simulink model "IEEE9Bus_new"  (R2020b)
settings: Solver=ode23tb  StartTime=0.0  StopTime=0.2  MaxStep=50e-6  RelTol=1e-3  EnableMultiTasking=on
values from neighbouring files (symbols this model uses):
  x = 50    [Xconst.m]    (also in wt_new.m = p(i))
libraries: powerlib x49
settings Model: Creator=salam  LastModifiedBy=Lenovo G50-80
settings DataIOCC: ReturnWorkspaceOutputs=off
settings DebuggingCC: ArithmeticOperatorsInVariantConditions=warning
settings SFSimCC: CustomCodeUndefinedFunction=UseInterfaceOnly
settings CodeAppCC: StateflowObjectComments=on
settings SimscapeCC: SimscapeNormalizeSystem=off

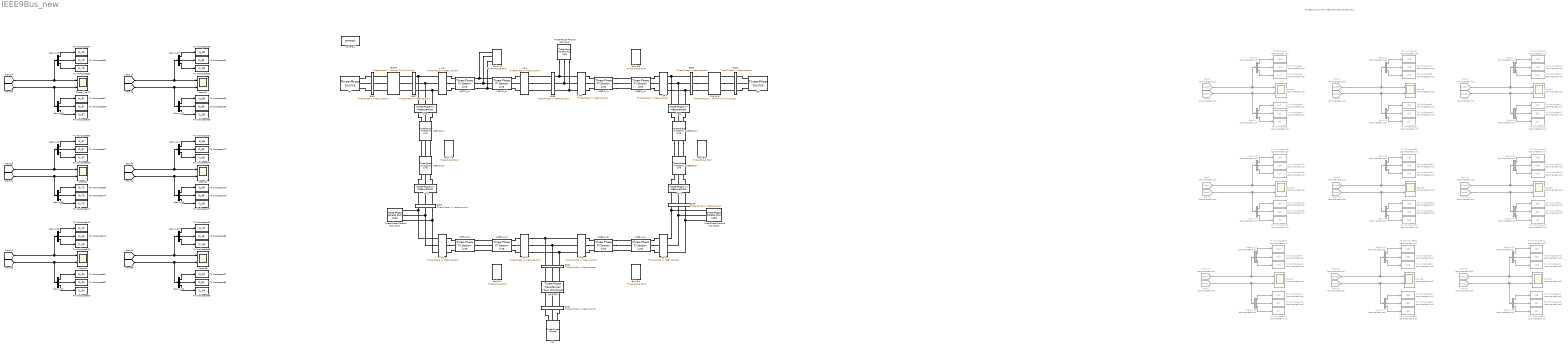
== system IEEE9Bus_new ==
  note: Voltage and Current Measurements at each Bus
  + 46 - : powerlib/Measurements/Three-Phase V-I Measurement  VoltageMeasurement=no  SetLabelV=on  LabelV=Vabc_78  Vpu=on  VpuLL=off  CurrentMeasurement=yes  SetLabelI=on  LabelI=Iabc_46  Ipu=off  Pbase=100e6  Vbase=230e3  OutputType=Complex  PhasorSimulation=off  PSBequivalent=0
  + 54 - : powerlib/Measurements/Three-Phase V-I Measurement  VoltageMeasurement=no  SetLabelV=on  LabelV=Vabc_78  Vpu=on  VpuLL=off  CurrentMeasurement=yes  SetLabelI=on  LabelI=Iabc_54  Ipu=off  Pbase=100e6  Vbase=230e3  OutputType=Complex  PhasorSimulation=off  PSBequivalent=0
  + 75 - : powerlib/Measurements/Three-Phase V-I Measurement  VoltageMeasurement=no  SetLabelV=on  LabelV=Vabc_87  Vpu=on  VpuLL=off  CurrentMeasurement=yes  SetLabelI=on  LabelI=Iabc_75  Ipu=off  Pbase=100e6  Vbase=230e3  OutputType=Complex  PhasorSimulation=off  PSBequivalent=0
  + 78 - : powerlib/Measurements/Three-Phase V-I Measurement  VoltageMeasurement=no  SetLabelV=on  LabelV=Vabc_78  Vpu=on  VpuLL=off  CurrentMeasurement=yes  SetLabelI=on  LabelI=Iabc_78  Ipu=off  Pbase=100e6  Vbase=230e3  OutputType=Complex  PhasorSimulation=off  PSBequivalent=0
  + 89 - : powerlib/Measurements/Three-Phase V-I Measurement  VoltageMeasurement=no  SetLabelV=on  LabelV=Vabc_78  Vpu=on  VpuLL=off  CurrentMeasurement=yes  SetLabelI=on  LabelI=Iabc_89  Ipu=off  Pbase=100e6  Vbase=230e3  OutputType=Complex  PhasorSimulation=off  PSBequivalent=0
  + 96 - : powerlib/Measurements/Three-Phase V-I Measurement  VoltageMeasurement=no  SetLabelV=on  LabelV=Vabc_87  Vpu=on  VpuLL=off  CurrentMeasurement=yes  SetLabelI=on  LabelI=Iabc_96  Ipu=off  Pbase=100e6  Vbase=230e3  OutputType=Complex  PhasorSimulation=off  PSBequivalent=0
  - 46 + : powerlib/Measurements/Three-Phase V-I Measurement  VoltageMeasurement=no  SetLabelV=on  LabelV=Vabc_87  Vpu=on  VpuLL=off  CurrentMeasurement=yes  SetLabelI=on  LabelI=Iabc_64  Ipu=off  Pbase=100e6  Vbase=230e3  OutputType=Complex  PhasorSimulation=off  PSBequivalent=0
  - 54 + : powerlib/Measurements/Three-Phase V-I Measurement  VoltageMeasurement=no  SetLabelV=on  LabelV=Vabc_87  Vpu=on  VpuLL=off  CurrentMeasurement=yes  SetLabelI=on  LabelI=Iabc_45  Ipu=off  Pbase=100e6  Vbase=230e3  OutputType=Complex  PhasorSimulation=off  PSBequivalent=0
  - 75 + : powerlib/Measurements/Three-Phase V-I Measurement  VoltageMeasurement=no  SetLabelV=on  LabelV=Vabc_87  Vpu=on  VpuLL=off  CurrentMeasurement=yes  SetLabelI=on  LabelI=Iabc_57  Ipu=off  Pbase=100e6  Vbase=230e3  OutputType=Complex  PhasorSimulation=off  PSBequivalent=0
  - 78 + : powerlib/Measurements/Three-Phase V-I Measurement  VoltageMeasurement=no  SetLabelV=on  LabelV=Vabc_87  Vpu=on  VpuLL=off  CurrentMeasurement=yes  SetLabelI=on  LabelI=Iabc_87  Ipu=off  Pbase=100e6  Vbase=230e3  OutputType=Complex  PhasorSimulation=off  PSBequivalent=0
  - 89 + : powerlib/Measurements/Three-Phase V-I Measurement  VoltageMeasurement=no  SetLabelV=on  LabelV=Vabc_87  Vpu=on  VpuLL=off  CurrentMeasurement=yes  SetLabelI=on  LabelI=Iabc_98  Ipu=off  Pbase=100e6  Vbase=230e3  OutputType=Complex  PhasorSimulation=off  PSBequivalent=0
  - 96 + : powerlib/Measurements/Three-Phase V-I Measurement  VoltageMeasurement=no  SetLabelV=on  LabelV=Vabc_87  Vpu=on  VpuLL=off  CurrentMeasurement=yes  SetLabelI=on  LabelI=Iabc_69  Ipu=off  Pbase=100e6  Vbase=230e3  OutputType=Complex  PhasorSimulation=off  PSBequivalent=0
  16.5/230 : powerlib/Elements/Three-Phase Transformer (Two Windings)  Winding1Connection=Yg  Winding2Connection=Yg  CoreType=Three single-phase transformers  SetSaturation=off  Hysteresis=off  DataFile='hysteresis'  SetInitialFlux=off  Measurements=None  UNITS=pu  NominalPower=[ 100e6 , 50 ]  Winding1=[ 24e3 , 1e-6, 0 ]  Winding2=[ 230e3 ,1e-6, 0.0576 ]  Rm=500  Lm=500  L0=0.5  Saturation=[ 0,0 ; 0.0024,1.2 ; 1.0,1.52 ]  InitialFluxes=[ 0.8 , -0.8 , 0.7 ]  BreakLoop=off  DiscreteSolver=Trapezoidal iterative  DataType=off  TransfoNumber=1
  18/230 : powerlib/Elements/Three-Phase Transformer (Two Windings)  Winding1Connection=Yg  Winding2Connection=Yg  CoreType=Three single-phase transformers  SetSaturation=off  Hysteresis=off  DataFile='hysteresis'  SetInitialFlux=off  Measurements=None  UNITS=pu  NominalPower=[ 100e6 , 50 ]  Winding1=[ 18e3 , 1e-6 , 0]  Winding2=[ 230e3 , 1e-6, 0.0625 ]  Rm=500  Lm=500  L0=0.5  Saturation=[ 0,0 ; 0.0024,1.2 ; 1.0,1.52 ]  InitialFluxes=[ 0.8 , -0.8 , 0.7 ]  BreakLoop=off  DiscreteSolver=Trapezoidal iterative  DataType=off  TransfoNumber=1
  230/13.8 : powerlib/Elements/Three-Phase Transformer (Two Windings)  Winding1Connection=Yg  Winding2Connection=Yg  CoreType=Three single-phase transformers  SetSaturation=off  Hysteresis=off  DataFile='hysteresis'  SetInitialFlux=off  Measurements=None  UNITS=pu  NominalPower=[ 100e6 , 50 ]  Winding1=[ 13.8e3 , 1e-6 , 0 ]  Winding2=[ 230e3 , 1e-6, 0.0586 ]  Rm=500  Lm=500  L0=0.5  Saturation=[ 0,0 ; 0.0024,1.2 ; 1.0,1.52 ]  InitialFluxes=[ 0.8 , -0.8 , 0.7 ]  BreakLoop=off  DiscreteSolver=Trapezoidal iterative  DataType=off  TransfoNumber=1
  BUS1 : powerlib/Measurements/Three-Phase V-I Measurement  VoltageMeasurement=phase-to-ground  SetLabelV=on  LabelV=Vabc1  Vpu=off  VpuLL=off  CurrentMeasurement=yes  SetLabelI=on  LabelI=Iabc1  Ipu=off  Pbase=100e6  Vbase=500e3  OutputType=Complex  PhasorSimulation=off  PSBequivalent=0
  BUS2 : powerlib/Measurements/Three-Phase V-I Measurement  VoltageMeasurement=phase-to-ground  SetLabelV=on  LabelV=Vabc2  Vpu=off  VpuLL=off  CurrentMeasurement=yes  SetLabelI=on  LabelI=Iabc2  Ipu=off  Pbase=100e6  Vbase=500e3  OutputType=Complex  PhasorSimulation=off  PSBequivalent=0
  BUS3 : powerlib/Measurements/Three-Phase V-I Measurement  VoltageMeasurement=phase-to-ground  SetLabelV=on  LabelV=Vabc3  Vpu=off  VpuLL=off  CurrentMeasurement=yes  SetLabelI=on  LabelI=Iabc3  Ipu=off  Pbase=100e6  Vbase=500e3  OutputType=Complex  PhasorSimulation=off  PSBequivalent=0
  BUS4 : powerlib/Measurements/Three-Phase V-I Measurement  VoltageMeasurement=phase-to-ground  SetLabelV=on  LabelV=Vabc4  Vpu=off  VpuLL=off  CurrentMeasurement=yes  SetLabelI=on  LabelI=Iabc4  Ipu=off  Pbase=100e6  Vbase=500e3  OutputType=Complex  PhasorSimulation=off  PSBequivalent=0
  BUS5 : powerlib/Measurements/Three-Phase V-I Measurement  VoltageMeasurement=phase-to-ground  SetLabelV=on  LabelV=Vabc5  Vpu=off  VpuLL=off  CurrentMeasurement=yes  SetLabelI=on  LabelI=Iabc5  Ipu=off  Pbase=100e6  Vbase=500e3  OutputType=Complex  PhasorSimulation=off  PSBequivalent=0
  BUS6 : powerlib/Measurements/Three-Phase V-I Measurement  VoltageMeasurement=phase-to-ground  SetLabelV=on  LabelV=Vabc6  Vpu=off  VpuLL=off  CurrentMeasurement=yes  SetLabelI=on  LabelI=Iabc6  Ipu=off  Pbase=100e6  Vbase=500e3  OutputType=Complex  PhasorSimulation=off  PSBequivalent=0
  BUS7 : powerlib/Measurements/Three-Phase V-I Measurement  VoltageMeasurement=phase-to-ground  SetLabelV=on  LabelV=Vabc7  Vpu=off  VpuLL=off  CurrentMeasurement=yes  SetLabelI=on  LabelI=Iabc7  Ipu=off  Pbase=100e6  Vbase=500e3  OutputType=Complex  PhasorSimulation=off  PSBequivalent=0
  BUS8 : powerlib/Measurements/Three-Phase V-I Measurement  VoltageMeasurement=phase-to-ground  SetLabelV=on  LabelV=Vabc8  Vpu=off  VpuLL=off  CurrentMeasurement=yes  SetLabelI=on  LabelI=Iabc8  Ipu=off  Pbase=100e6  Vbase=500e3  OutputType=Complex  PhasorSimulation=off  PSBequivalent=0
  BUS9 : powerlib/Measurements/Three-Phase V-I Measurement  VoltageMeasurement=phase-to-ground  SetLabelV=on  LabelV=Vabc9  Vpu=off  VpuLL=off  CurrentMeasurement=yes  SetLabelI=on  LabelI=Iabc9  Ipu=off  Pbase=100e6  Vbase=500e3  OutputType=Complex  PhasorSimulation=off  PSBequivalent=0
  Demux{,1..17} (18 alike) : Demux  Commented=on  Outputs=3
  Demux{18..29} (12 alike) : Demux  Outputs=3
  From1 : From  Commented=on  GotoTag=Vabc1  TagVisibility=global
  From10 : From  Commented=on  GotoTag=Iabc5  TagVisibility=global
  From11 : From  Commented=on  GotoTag=Vabc6  TagVisibility=global
  From12 : From  Commented=on  GotoTag=Iabc6  TagVisibility=global
  From13 : From  Commented=on  GotoTag=Iabc8  TagVisibility=global
  From14 : From  Commented=on  GotoTag=Vabc9  TagVisibility=global
  From15 : From  Commented=on  GotoTag=Iabc9  TagVisibility=global
  From16 : From  Commented=on  GotoTag=Vabc7  TagVisibility=global
  From17 : From  Commented=on  GotoTag=Iabc7  TagVisibility=global
  From18 : From  Commented=on  GotoTag=Vabc8  TagVisibility=global
  From2 : From  Commented=on  GotoTag=Iabc1  TagVisibility=global
  From3 : From  Commented=on  GotoTag=Vabc2  TagVisibility=global
  From4 : From  Commented=on  GotoTag=Iabc2  TagVisibility=global
  From5 : From  Commented=on  GotoTag=Vabc3  TagVisibility=global
  From6 : From  Commented=on  GotoTag=Iabc3  TagVisibility=global
  From7 : From  Commented=on  GotoTag=Vabc4  TagVisibility=global
  From8 : From  Commented=on  GotoTag=Iabc4  TagVisibility=global
  From9 : From  Commented=on  GotoTag=Vabc5  TagVisibility=global
  G1 : powerlib/Electrical Sources/Three-Phase Source  InternalConnection=Yg  VoltagePhases=off  Voltage=16500  PhaseAngle=0  Voltage_phases=[25e3 25e3 25e3]/sqrt(3)  PhaseAngles_phases=[0 -120 +120]  Frequency=50  NonIdealSource=on  SpecifyImpedance=off  Resistance=0.8929  Inductance=16.58e-3  ShortCircuitLevel=247.5e6  BaseVoltage=16.5e3  XRratio=100000  BusType=swing  Pref=10e3  Qref=0  Prefabc=[10e3, 10e3, 10e3]  Qrefabc=[0, 0, 0]  Qmin=-inf  Qmax=inf
  G2 : powerlib/Electrical Sources/Three-Phase Source  InternalConnection=Yg  VoltagePhases=off  Voltage=18e3  PhaseAngle=0  Voltage_phases=[25e3 25e3 25e3]/sqrt(3)  PhaseAngles_phases=[0 -120 +120]  Frequency=50  NonIdealSource=on  SpecifyImpedance=off  Resistance=0.8929  Inductance=16.58e-3  ShortCircuitLevel=192e6  BaseVoltage=18e3  XRratio=100000  BusType=PV  Pref=163e6  Qref=0  Prefabc=[10e3, 10e3, 10e3]  Qrefabc=[0, 0, 0]  Qmin=-inf  Qmax=inf
  G3 : powerlib/Electrical Sources/Three-Phase Source  InternalConnection=Yg  VoltagePhases=off  Voltage=13800  PhaseAngle=0  Voltage_phases=[25e3 25e3 25e3]/sqrt(3)  PhaseAngles_phases=[0 -120 +120]  Frequency=50  NonIdealSource=on  SpecifyImpedance=off  Resistance=0.8929  Inductance=16.58e-3  ShortCircuitLevel=128e6  BaseVoltage=13.8e3  XRratio=100000  BusType=PV  Pref=85e6  Qref=0  Prefabc=[10e3, 10e3, 10e3]  Qrefabc=[0, 0, 0]  Qmin=-inf  Qmax=inf
  LINE5-4_(1) : powerlib/Elements/Three-Phase PI Section Line  LConnTagsString=a|b|c  RConnTagsString=A|B|C  Length=47.38  Frequency=50  Resistances=[ 0.01273 0.3864]  Inductances="[ 0.9337e-3  4.1264e-3]"  Capacitances=[12.74e-9 7.751e-9]
  LINE5-4_(2) : powerlib/Elements/Three-Phase PI Section Line  LConnTagsString=a|b|c  RConnTagsString=A|B|C  Length=50  Frequency=50  Resistances=[ 0.01273 0.3864]  Inductances="[ 0.9337e-3  4.1264e-3]"  Capacitances=[12.74e-9 7.751e-9]
  LINE6-4_(1) : powerlib/Elements/Three-Phase PI Section Line  LConnTagsString=a|b|c  RConnTagsString=A|B|C  Length=45.99  Frequency=50  Resistances=[ 0.01273 0.3864]  Inductances="[ 0.9337e-3  4.1264e-3]"  Capacitances=[12.74e-9 7.751e-9]
  LINE6-4_(2) : powerlib/Elements/Three-Phase PI Section Line  LConnTagsString=a|b|c  RConnTagsString=A|B|C  Length=50  Frequency=50  Resistances=[ 0.01273 0.3864]  Inductances="[ 0.9337e-3  4.1264e-3]"  Capacitances=[12.74e-9 7.751e-9]
  LINE7-5_(1) : powerlib/Elements/Three-Phase PI Section Line  LConnTagsString=a|b|c  RConnTagsString=A|B|C  Length=100  Frequency=50  Resistances=[ 0.01273 0.3864]  Inductances="[ 0.9337e-3  4.1264e-3]"  Capacitances=[12.74e-9 7.751e-9]
  LINE7-5_(2) : powerlib/Elements/Three-Phase PI Section Line  LConnTagsString=a|b|c  RConnTagsString=A|B|C  Length=76.71  Frequency=50  Resistances=[ 0.01273 0.3864]  Inductances="[ 0.9337e-3  4.1264e-3]"  Capacitances=[12.74e-9 7.751e-9]
  LINE7-8_(1) : powerlib/Elements/Three-Phase PI Section Line  LConnTagsString=a|b|c  RConnTagsString=A|B|C  Length=98.95*x*.01+.001  Frequency=50  Resistances=[ 0.01273 0.3864]  Inductances="[ 0.9337e-3  4.1264e-3]"  Capacitances=[12.74e-9 7.751e-9]
  LINE7-8_(2) : powerlib/Elements/Three-Phase PI Section Line  LConnTagsString=a|b|c  RConnTagsString=A|B|C  Length=98.95*(1-x*.01)+.001  Frequency=50  Resistances=[ 0.01273 0.3864]  Inductances="[ 0.9337e-3  4.1264e-3]"  Capacitances=[12.74e-9 7.751e-9]
  LINE8-9_(1) : powerlib/Elements/Three-Phase PI Section Line  LConnTagsString=a|b|c  RConnTagsString=A|B|C  Length=65.56  Frequency=50  Resistances=[ 0.01273 0.3864]  Inductances="[ 0.9337e-3  4.1264e-3]"  Capacitances=[12.74e-9 7.751e-9]
  LINE8-9_(2) : powerlib/Elements/Three-Phase PI Section Line  LConnTagsString=a|b|c  RConnTagsString=A|B|C  Length=50  Frequency=50  Resistances=[ 0.01273 0.3864]  Inductances="[ 0.9337e-3  4.1264e-3]"  Capacitances=[12.74e-9 7.751e-9]
  LINE9-6_(1) : powerlib/Elements/Three-Phase PI Section Line  LConnTagsString=a|b|c  RConnTagsString=A|B|C  Length=100  Frequency=50  Resistances=[ 0.01273 0.3864]  Inductances="[ 0.9337e-3  4.1264e-3]"  Capacitances=[12.74e-9 7.751e-9]
  LINE9-6_(2) : powerlib/Elements/Three-Phase PI Section Line  LConnTagsString=a|b|c  RConnTagsString=A|B|C  Length=96.41  Frequency=50  Resistances=[ 0.01273 0.3864]  Inductances="[ 0.9337e-3  4.1264e-3]"  Capacitances=[12.74e-9 7.751e-9]
  Scope{1..9} (9 alike) : Scope  Commented=on  NumInputPorts=2
  Scope{11..15} (5 alike) : Scope  NumInputPorts=2
  Scope_line78 : Scope  NumInputPorts=2
  Three-Phase Parallel RLC Load : powerlib/Elements/Three-Phase Parallel RLC Load  LConnTagsString=A|B|C  Configuration=Y (grounded)  NominalVoltage=230000  Vabc=[1e3 1e3 1e3]  Vabcp=[1e3 1e3 1e3]  NominalFrequency=50  UnbalancedPower=off  ActivePower=100e6  InductivePower=35e6  CapacitivePower=0  Pabc=[10e3 9e3 11e3]  QLabc=[100 90 110]  QCabc=[100 90 110]  Pabcp=[10e3 9e3 11e3]  QLabcp=[100 90 110]  QCabcp=[100 90 110]  Measurements=None  LoadType=constant Z
  Three-Phase Parallel RLC Load1 : powerlib/Elements/Three-Phase Parallel RLC Load  LConnTagsString=A|B|C  Configuration=Y (grounded)  NominalVoltage=230000  Vabc=[1e3 1e3 1e3]  Vabcp=[1e3 1e3 1e3]  NominalFrequency=50  UnbalancedPower=off  ActivePower=125e6  InductivePower=50e6  CapacitivePower=0  Pabc=[10e3 9e3 11e3]  QLabc=[100 90 110]  QCabc=[100 90 110]  Pabcp=[10e3 9e3 11e3]  QLabcp=[100 90 110]  QCabcp=[100 90 110]  Measurements=None  LoadType=constant Z
  Three-Phase Parallel RLC Load2 : powerlib/Elements/Three-Phase Parallel RLC Load  LConnTagsString=A|B|C  Configuration=Y (grounded)  NominalVoltage=230000  Vabc=[1e3 1e3 1e3]  Vabcp=[1e3 1e3 1e3]  NominalFrequency=50  UnbalancedPower=off  ActivePower=90e6  InductivePower=30e6  CapacitivePower=0  Pabc=[10e3 9e3 11e3]  QLabc=[100 90 110]  QCabc=[100 90 110]  Pabcp=[10e3 9e3 11e3]  QLabcp=[100 90 110]  QCabcp=[100 90 110]  Measurements=None  LoadType=constant Z
  To Workspace : ToWorkspace  Commented=on  VariableName=Va1  SampleTime=-1
  To Workspace1 : ToWorkspace  Commented=on  VariableName=Vb1  SampleTime=-1
  To Workspace10 : ToWorkspace  Commented=on  VariableName=Ib2  SampleTime=-1
  To Workspace11 : ToWorkspace  Commented=on  VariableName=Ic2  SampleTime=-1
  To Workspace12 : ToWorkspace  Commented=on  VariableName=Ib3  SampleTime=-1
  To Workspace13 : ToWorkspace  Commented=on  VariableName=Ic3  SampleTime=-1
  To Workspace14 : ToWorkspace  Commented=on  VariableName=Va3  SampleTime=-1
  To Workspace15 : ToWorkspace  Commented=on  VariableName=Vb3  SampleTime=-1
  To Workspace16 : ToWorkspace  Commented=on  VariableName=Vc3  SampleTime=-1
  To Workspace17 : ToWorkspace  Commented=on  VariableName=Ia3  SampleTime=-1
  To Workspace18 : ToWorkspace  Commented=on  VariableName=Va4  SampleTime=-1
  To Workspace19 : ToWorkspace  Commented=on  VariableName=Vb4  SampleTime=-1
  To Workspace2 : ToWorkspace  Commented=on  VariableName=Vc1  SampleTime=-1
  To Workspace20 : ToWorkspace  Commented=on  VariableName=Ib5  SampleTime=-1
  To Workspace21 : ToWorkspace  Commented=on  VariableName=Ic5  SampleTime=-1
  To Workspace22 : ToWorkspace  Commented=on  VariableName=Ib6  SampleTime=-1
  To Workspace23 : ToWorkspace  Commented=on  VariableName=Ic6  SampleTime=-1
  To Workspace24 : ToWorkspace  Commented=on  VariableName=Va6  SampleTime=-1
  To Workspace25 : ToWorkspace  Commented=on  VariableName=Vb6  SampleTime=-1
  To Workspace26 : ToWorkspace  Commented=on  VariableName=Vc6  SampleTime=-1
  To Workspace27 : ToWorkspace  Commented=on  VariableName=Ia6  SampleTime=-1
  To Workspace28 : ToWorkspace  Commented=on  VariableName=Vc4  SampleTime=-1
  To Workspace29 : ToWorkspace  Commented=on  VariableName=Ia4  SampleTime=-1
  To Workspace3 : ToWorkspace  Commented=on  VariableName=Ia1  SampleTime=-1
  To Workspace30 : ToWorkspace  Commented=on  VariableName=Ib4  SampleTime=-1
  To Workspace31 : ToWorkspace  Commented=on  VariableName=Ic4  SampleTime=-1
  To Workspace32 : ToWorkspace  Commented=on  VariableName=Va5  SampleTime=-1
  To Workspace33 : ToWorkspace  Commented=on  VariableName=Vb5  SampleTime=-1
  To Workspace34 : ToWorkspace  Commented=on  VariableName=Vc5  SampleTime=-1
  To Workspace35 : ToWorkspace  Commented=on  VariableName=Ia5  SampleTime=-1
  To Workspace36 : ToWorkspace  Commented=on  VariableName=Va7  SampleTime=-1
  To Workspace37 : ToWorkspace  Commented=on  VariableName=Vb7  SampleTime=-1
  To Workspace38 : ToWorkspace  Commented=on  VariableName=Ib8  SampleTime=-1
  To Workspace39 : ToWorkspace  Commented=on  VariableName=Ic8  SampleTime=-1
  To Workspace4 : ToWorkspace  Commented=on  VariableName=Ib1  SampleTime=-1
  To Workspace40 : ToWorkspace  Commented=on  VariableName=Ib9  SampleTime=-1
  To Workspace41 : ToWorkspace  Commented=on  VariableName=Ic9  SampleTime=-1
  To Workspace42 : ToWorkspace  Commented=on  VariableName=Va9  SampleTime=-1
  To Workspace43 : ToWorkspace  Commented=on  VariableName=Vb9  SampleTime=-1
  To Workspace44 : ToWorkspace  Commented=on  VariableName=Vc9  SampleTime=-1
  To Workspace45 : ToWorkspace  Commented=on  VariableName=Ia9  SampleTime=-1
  To Workspace46 : ToWorkspace  Commented=on  VariableName=Vc7  SampleTime=-1
  To Workspace47 : ToWorkspace  Commented=on  VariableName=Ia7  SampleTime=-1
  To Workspace48 : ToWorkspace  Commented=on  VariableName=Ib7  SampleTime=-1
  To Workspace49 : ToWorkspace  Commented=on  VariableName=Ic7  SampleTime=-1
  To Workspace5 : ToWorkspace  Commented=on  VariableName=Ic1  SampleTime=-1
  To Workspace50 : ToWorkspace  Commented=on  VariableName=Va8  SampleTime=-1
  To Workspace51 : ToWorkspace  Commented=on  VariableName=Vb8  SampleTime=-1
  To Workspace52 : ToWorkspace  Commented=on  VariableName=Vc8  SampleTime=-1
  To Workspace53 : ToWorkspace  Commented=on  VariableName=Ia8  SampleTime=-1
  To Workspace54 : ToWorkspace  VariableName=Ia_78  SampleTime=-1
  To Workspace55 : ToWorkspace  VariableName=Ib_78  SampleTime=-1
  To Workspace56 : ToWorkspace  VariableName=Ic_78  SampleTime=-1
  To Workspace57 : ToWorkspace  VariableName=Ia_87  SampleTime=-1
  To Workspace58 : ToWorkspace  VariableName=Ib_87  SampleTime=-1
  To Workspace59 : ToWorkspace  VariableName=Ic_87  SampleTime=-1
  To Workspace6 : ToWorkspace  Commented=on  VariableName=Va2  SampleTime=-1
  To Workspace60 : ToWorkspace  VariableName=Ia_89  SampleTime=-1
  To Workspace61 : ToWorkspace  VariableName=Ib_89  SampleTime=-1
  To Workspace62 : ToWorkspace  VariableName=Ic_89  SampleTime=-1
  To Workspace63 : ToWorkspace  VariableName=Ia_98  SampleTime=-1
  To Workspace64 : ToWorkspace  VariableName=Ib_98  SampleTime=-1
  To Workspace65 : ToWorkspace  VariableName=Ic_98  SampleTime=-1
  To Workspace66 : ToWorkspace  VariableName=Ia_57  SampleTime=-1
  To Workspace67 : ToWorkspace  VariableName=Ib_57  SampleTime=-1
  To Workspace68 : ToWorkspace  VariableName=Ic_57  SampleTime=-1
  To Workspace69 : ToWorkspace  VariableName=Ia_75  SampleTime=-1
  To Workspace7 : ToWorkspace  Commented=on  VariableName=Vb2  SampleTime=-1
  To Workspace70 : ToWorkspace  VariableName=Ib_75  SampleTime=-1
  To Workspace71 : ToWorkspace  VariableName=Ic_75  SampleTime=-1
  To Workspace72 : ToWorkspace  VariableName=Ia_69  SampleTime=-1
  To Workspace73 : ToWorkspace  VariableName=Ib_69  SampleTime=-1
  To Workspace74 : ToWorkspace  VariableName=Ic_69  SampleTime=-1
  To Workspace75 : ToWorkspace  VariableName=Ia_96  SampleTime=-1
  To Workspace76 : ToWorkspace  VariableName=Ib_96  SampleTime=-1
  To Workspace77 : ToWorkspace  VariableName=Ic_96  SampleTime=-1
  To Workspace78 : ToWorkspace  VariableName=Ia_45  SampleTime=-1
  To Workspace79 : ToWorkspace  VariableName=Ib_45  SampleTime=-1
  To Workspace8 : ToWorkspace  Commented=on  VariableName=Vc2  SampleTime=-1
  To Workspace80 : ToWorkspace  VariableName=Ic_45  SampleTime=-1
  To Workspace81 : ToWorkspace  VariableName=Ia_54  SampleTime=-1
  To Workspace82 : ToWorkspace  VariableName=Ib_54  SampleTime=-1
  To Workspace83 : ToWorkspace  VariableName=Ic_54  SampleTime=-1
  To Workspace84 : ToWorkspace  VariableName=Ia_46  SampleTime=-1
  To Workspace85 : ToWorkspace  VariableName=Ib_46  SampleTime=-1
  To Workspace86 : ToWorkspace  VariableName=Ic_46  SampleTime=-1
  To Workspace87 : ToWorkspace  VariableName=Ia_64  SampleTime=-1
  To Workspace88 : ToWorkspace  VariableName=Ib_64  SampleTime=-1
  To Workspace89 : ToWorkspace  VariableName=Ic_64  SampleTime=-1
  To Workspace9 : ToWorkspace  Commented=on  VariableName=Ia2  SampleTime=-1
  fault 5-4 : powerlib/Elements/Three-Phase Fault  InitialStates=0  FaultA=on  FaultB=off  FaultC=off  GroundFault=on  SwitchTimes=[2/50 8/50]  External=off  SwitchStatus=NaN  FaultResistance=0.001  GroundResistance=0.01  SnubberResistance=1e6  SnubberCapacitance=inf  Measurements=None
  fault 6-4 : powerlib/Elements/Three-Phase Fault  InitialStates=0  FaultA=on  FaultB=off  FaultC=off  GroundFault=on  SwitchTimes=[2/50 8/50]  External=off  SwitchStatus=NaN  FaultResistance=0.001  GroundResistance=0.01  SnubberResistance=1e6  SnubberCapacitance=inf  Measurements=None
  fault 6-9 : powerlib/Elements/Three-Phase Fault  InitialStates=0  FaultA=on  FaultB=off  FaultC=off  GroundFault=on  SwitchTimes=[2/50 8/50]  External=off  SwitchStatus=NaN  FaultResistance=0.001  GroundResistance=0.01  SnubberResistance=1e6  SnubberCapacitance=inf  Measurements=None
  fault 7-5 : powerlib/Elements/Three-Phase Fault  InitialStates=0  FaultA=on  FaultB=off  FaultC=off  GroundFault=on  SwitchTimes=[2/50 8/50]  External=off  SwitchStatus=NaN  FaultResistance=0.001  GroundResistance=0.01  SnubberResistance=1e6  SnubberCapacitance=inf  Measurements=None
  "fault 7-8 " : powerlib/Elements/Three-Phase Fault  InitialStates=0  FaultA=on  FaultB=off  FaultC=off  GroundFault=on  SwitchTimes=[2/50 8/50]  External=off  SwitchStatus=NaN  FaultResistance=0.01  GroundResistance=0.01  SnubberResistance=1e6  SnubberCapacitance=inf  Measurements=None
  fault 8-9 : powerlib/Elements/Three-Phase Fault  InitialStates=0  FaultA=on  FaultB=off  FaultC=off  GroundFault=on  SwitchTimes=[2/50 8/50]  External=off  SwitchStatus=NaN  FaultResistance=0.001  GroundResistance=0.01  SnubberResistance=1e6  SnubberCapacitance=inf  Measurements=None
  powergui : powerlib/powergui  Priority=1  SimulationMode=Discrete  SampleTime=50e-6  frequency=60  Iterations=50  frequencyindice=0  Pbase=100e6  ErrMax=1e-4  UnitsV=kV  UnitsW=MW  buscounter=0  FunctionMessages=off  echomessages=off  EnableUseOfTLC=off  CurrentSourceSwitches=off  DisableSnubberDevices=off  DisableRonSwitches=off  DisableVfSwitches=off  DisplayEquations=off  AutomaticDiscreteSolvers=off  SolverType=Tustin/Backward Euler (TBE)  Interpol=off  ExternalGateDelay=off  methode=off  Ts=100  x0status=blocks  SPID=on  SwTol=0  HookPort=off  NonlinearTolerance=1e-4  nMaxIteration=100  ContinueOnMaxIteration=off  RestoreLinks=warning  ResistiveCurrentMeasurement=off  Frange=[0:2:500]  Ylog=off  Xlog=on  ShowGrid=off  save=off  variable=ZData  structure=0  ZoomFFT=off  StartTime=0.0  cycles=1  DisplayStyle=1  fundamental=60  FreqAxis=off  MaxFrequency=1000  frequencyindicesteady=1  RmsSteady=1  display=off
  wires:
  From1/1 -> Demux/1, Scope1/1
  Demux/2 -> To Workspace1/1
  Demux/1 -> To Workspace/1
  Demux/3 -> To Workspace2/1
  Demux1/3 -> To Workspace5/1
  Demux1/1 -> To Workspace3/1
  Demux1/2 -> To Workspace4/1
  From2/1 -> Demux1/1, Scope1/2
  From4/1 -> Scope2/2, Demux3/1
  Demux3/2 -> To Workspace10/1
  Demux3/1 -> To Workspace9/1
  Demux3/3 -> To Workspace11/1
  Demux2/3 -> To Workspace8/1
  Demux2/1 -> To Workspace6/1
  Demux2/2 -> To Workspace7/1
  From3/1 -> Scope2/1, Demux2/1
  From5/1 -> Demux4/1, Scope3/1
  Demux4/2 -> To Workspace15/1
  Demux4/1 -> To Workspace14/1
  Demux4/3 -> To Workspace16/1
  Demux5/3 -> To Workspace13/1
  Demux5/1 -> To Workspace17/1
  Demux5/2 -> To Workspace12/1
  From6/1 -> Demux5/1, Scope3/2
  From12/1 -> Scope6/2, Demux11/1
  Demux11/2 -> To Workspace22/1
  Demux11/1 -> To Workspace27/1
  Demux11/3 -> To Workspace23/1
  Demux10/3 -> To Workspace26/1
  Demux10/1 -> To Workspace24/1
  Demux10/2 -> To Workspace25/1
  From11/1 -> Scope6/1, Demux10/1
  From9/1 -> Demux8/1, Scope5/1
  Demux8/2 -> To Workspace33/1
  Demux8/1 -> To Workspace32/1
  Demux8/3 -> To Workspace34/1
  Demux9/3 -> To Workspace21/1
  Demux9/1 -> To Workspace35/1
  Demux9/2 -> To Workspace20/1
  From10/1 -> Demux9/1, Scope5/2
  From8/1 -> Scope4/2, Demux7/1
  Demux7/2 -> To Workspace30/1
  Demux7/1 -> To Workspace29/1
  Demux7/3 -> To Workspace31/1
  Demux6/3 -> To Workspace28/1
  Demux6/1 -> To Workspace18/1
  Demux6/2 -> To Workspace19/1
  From7/1 -> Scope4/1, Demux6/1
  From16/1 -> Demux14/1, Scope7/1
  Demux14/2 -> To Workspace37/1
  Demux14/1 -> To Workspace36/1
  Demux14/3 -> To Workspace46/1
  Demux15/3 -> To Workspace49/1
  Demux15/1 -> To Workspace47/1
  Demux15/2 -> To Workspace48/1
  From17/1 -> Demux15/1, Scope7/2
  From13/1 -> Scope8/2, Demux17/1
  Demux17/2 -> To Workspace38/1
  Demux17/1 -> To Workspace53/1
  Demux17/3 -> To Workspace39/1
  Demux16/3 -> To Workspace52/1
  Demux16/1 -> To Workspace50/1
  Demux16/2 -> To Workspace51/1
  From18/1 -> Scope8/1, Demux16/1
  From14/1 -> Demux12/1, Scope9/1
  Demux12/2 -> To Workspace43/1
  Demux12/1 -> To Workspace42/1
  Demux12/3 -> To Workspace44/1
  Demux13/3 -> To Workspace41/1
  Demux13/1 -> To Workspace45/1
  Demux13/2 -> To Workspace40/1
  From15/1 -> Demux13/1, Scope9/2
  [Iabc_87] -> Scope_line78/2, Demux19/1
  Demux19/2 -> To Workspace58/1
  Demux19/1 -> To Workspace57/1
  Demux19/3 -> To Workspace59/1
  Demux18/3 -> To Workspace56/1
  Demux18/1 -> To Workspace54/1
  Demux18/2 -> To Workspace55/1
  [Iabc_78] -> Scope_line78/1, Demux18/1
  [Iabc_89] -> Demux20/1, Scope11/1
  Demux20/2 -> To Workspace61/1
  Demux20/1 -> To Workspace60/1
  Demux20/3 -> To Workspace62/1
  Demux21/3 -> To Workspace65/1
  Demux21/1 -> To Workspace63/1
  Demux21/2 -> To Workspace64/1
  [Iabc_98] -> Demux21/1, Scope11/2
  [Iabc_96] -> Scope13/2, Demux25/1
  Demux25/2 -> To Workspace76/1
  Demux25/1 -> To Workspace75/1
  Demux25/3 -> To Workspace77/1
  Demux24/3 -> To Workspace74/1
  Demux24/1 -> To Workspace72/1
  Demux24/2 -> To Workspace73/1
  [Iabc_69] -> Scope13/1, Demux24/1
  [Iabc_57] -> Demux22/1, Scope12/1
  Demux22/2 -> To Workspace67/1
  Demux22/1 -> To Workspace66/1
  Demux22/3 -> To Workspace68/1
  Demux23/3 -> To Workspace71/1
  Demux23/1 -> To Workspace69/1
  Demux23/2 -> To Workspace70/1
  [Iabc_75] -> Demux23/1, Scope12/2
  [Iabc_54] -> Scope14/2, Demux27/1
  Demux27/2 -> To Workspace82/1
  Demux27/1 -> To Workspace81/1
  Demux27/3 -> To Workspace83/1
  Demux26/3 -> To Workspace80/1
  Demux26/1 -> To Workspace78/1
  Demux26/2 -> To Workspace79/1
  [Iabc_45] -> Scope14/1, Demux26/1
  [Iabc_46] -> Demux28/1, Scope15/1
  Demux28/2 -> To Workspace85/1
  Demux28/1 -> To Workspace84/1
  Demux28/3 -> To Workspace86/1
  Demux29/3 -> To Workspace89/1
  Demux29/1 -> To Workspace87/1
  Demux29/2 -> To Workspace88/1
  [Iabc_64] -> Demux29/1, Scope15/2
  connections:
  BUS2/LConn1 -- G2/RConn1
  BUS2/LConn2 -- G2/RConn2
  BUS2/LConn3 -- G2/RConn3
  BUS2/RConn1 -- 18/230/LConn1
  BUS2/RConn2 -- 18/230/LConn2
  BUS2/RConn3 -- 18/230/LConn3
  BUS7/LConn3 -- 18/230/RConn3
  BUS7/LConn1 -- 18/230/RConn1
  18/230/RConn2 -- BUS7/LConn2
  BUS1/RConn1 -- 16.5/230/LConn1
  G1/RConn2 -- BUS1/LConn2
  BUS1/RConn2 -- 16.5/230/LConn2
  G1/RConn3 -- BUS1/LConn3
  G1/RConn1 -- BUS1/LConn1
  BUS1/RConn3 -- 16.5/230/LConn3
  16.5/230/RConn1 -- BUS4/LConn1
  16.5/230/RConn2 -- BUS4/LConn2
  BUS4/LConn3 -- 16.5/230/RConn3
  LINE7-5_(2)/LConn1 -- LINE7-5_(1)/RConn1
  LINE7-5_(2)/LConn2 -- LINE7-5_(1)/RConn2
  LINE7-5_(2)/LConn3 -- LINE7-5_(1)/RConn3
  LINE9-6_(1)/RConn1 -- LINE9-6_(2)/LConn1
  LINE9-6_(1)/RConn2 -- LINE9-6_(2)/LConn2
  LINE9-6_(1)/RConn3 -- LINE9-6_(2)/LConn3
  LINE6-4_(2)/LConn1 -- LINE6-4_(1)/RConn1
  LINE6-4_(2)/LConn2 -- LINE6-4_(1)/RConn2
  LINE6-4_(2)/LConn3 -- LINE6-4_(1)/RConn3
  LINE5-4_(1)/LConn1 -- LINE5-4_(2)/RConn1
  LINE5-4_(1)/LConn2 -- LINE5-4_(2)/RConn2
  LINE5-4_(1)/LConn3 -- LINE5-4_(2)/RConn3
  LINE7-8_(1)/RConn1 -- "fault 7-8 "/LConn1 -- LINE7-8_(2)/LConn1
  LINE7-8_(1)/RConn2 -- "fault 7-8 "/LConn2 -- LINE7-8_(2)/LConn2
  LINE7-8_(1)/RConn3 -- "fault 7-8 "/LConn3 -- LINE7-8_(2)/LConn3
  + 78 -/RConn1 -- LINE7-8_(1)/LConn1
  + 78 -/RConn2 -- LINE7-8_(1)/LConn2
  + 78 -/RConn3 -- LINE7-8_(1)/LConn3
  - 78 +/RConn1 -- LINE7-8_(2)/RConn1
  - 78 +/RConn2 -- LINE7-8_(2)/RConn2
  - 78 +/RConn3 -- LINE7-8_(2)/RConn3
  BUS7/RConn1 -- + 78 -/LConn1 -- + 75 -/LConn1
  BUS7/RConn2 -- + 78 -/LConn2 -- + 75 -/LConn2
  BUS7/RConn3 -- + 75 -/LConn3 -- + 78 -/LConn3
  - 78 +/LConn1 -- BUS8/LConn1
  - 78 +/LConn2 -- BUS8/LConn2
  - 78 +/LConn3 -- BUS8/LConn3
  + 54 -/RConn1 -- LINE5-4_(1)/RConn1
  + 54 -/RConn2 -- LINE5-4_(1)/RConn2
  + 54 -/RConn3 -- LINE5-4_(1)/RConn3
  LINE5-4_(2)/LConn1 -- - 54 +/RConn1
  LINE5-4_(2)/LConn2 -- - 54 +/RConn2
  LINE5-4_(2)/LConn3 -- - 54 +/RConn3
  BUS5/LConn3 -- + 54 -/LConn3 -- Three-Phase Parallel RLC Load1/LConn3
  BUS5/LConn1 -- Three-Phase Parallel RLC Load1/LConn1 -- + 54 -/LConn1
  BUS5/LConn2 -- Three-Phase Parallel RLC Load1/LConn2 -- + 54 -/LConn2
  LINE8-9_(1)/RConn1 -- LINE8-9_(2)/LConn1
  LINE8-9_(1)/RConn2 -- LINE8-9_(2)/LConn2
  LINE8-9_(1)/RConn3 -- LINE8-9_(2)/LConn3
  + 89 -/LConn1 -- BUS8/RConn1 -- Three-Phase Parallel RLC Load/LConn1
  + 89 -/LConn2 -- BUS8/RConn2 -- Three-Phase Parallel RLC Load/LConn2
  + 89 -/LConn3 -- BUS8/RConn3 -- Three-Phase Parallel RLC Load/LConn3
  + 89 -/RConn2 -- LINE8-9_(1)/LConn2
  + 89 -/RConn1 -- LINE8-9_(1)/LConn1
  + 89 -/RConn3 -- LINE8-9_(1)/LConn3
  LINE8-9_(2)/RConn1 -- - 89 +/RConn1
  LINE8-9_(2)/RConn2 -- - 89 +/RConn2
  LINE8-9_(2)/RConn3 -- - 89 +/RConn3
  - 54 +/LConn1 -- BUS4/RConn1 -- + 46 -/LConn1
  - 54 +/LConn2 -- BUS4/RConn2 -- + 46 -/LConn2
  - 54 +/LConn3 -- BUS4/RConn3 -- + 46 -/LConn3
  + 46 -/RConn1 -- LINE6-4_(2)/RConn1
  + 46 -/RConn2 -- LINE6-4_(2)/RConn2
  + 46 -/RConn3 -- LINE6-4_(2)/RConn3
  LINE6-4_(1)/LConn1 -- - 46 +/RConn1
  LINE6-4_(1)/LConn2 -- - 46 +/RConn2
  LINE6-4_(1)/LConn3 -- - 46 +/RConn3
  - 46 +/LConn1 -- Three-Phase Parallel RLC Load2/LConn1 -- BUS6/LConn1
  BUS6/LConn2 -- Three-Phase Parallel RLC Load2/LConn2 -- - 46 +/LConn2
  BUS6/LConn3 -- - 46 +/LConn3 -- Three-Phase Parallel RLC Load2/LConn3
  + 75 -/RConn1 -- LINE7-5_(1)/LConn1
  + 75 -/RConn2 -- LINE7-5_(1)/LConn2
  + 75 -/RConn3 -- LINE7-5_(1)/LConn3
  - 75 +/RConn1 -- LINE7-5_(2)/RConn1
  - 75 +/RConn2 -- LINE7-5_(2)/RConn2
  - 75 +/RConn3 -- LINE7-5_(2)/RConn3
  BUS5/RConn1 -- - 75 +/LConn1
  BUS5/RConn2 -- - 75 +/LConn2
  BUS5/RConn3 -- - 75 +/LConn3
  LINE9-6_(1)/LConn2 -- + 96 -/RConn2
  + 96 -/RConn1 -- LINE9-6_(1)/LConn1
  + 96 -/RConn3 -- LINE9-6_(1)/LConn3
  BUS6/RConn1 -- - 96 +/LConn1
  BUS6/RConn2 -- - 96 +/LConn2
  BUS6/RConn3 -- - 96 +/LConn3
  - 96 +/RConn2 -- LINE9-6_(2)/RConn2
  - 96 +/RConn1 -- LINE9-6_(2)/RConn1
  - 96 +/RConn3 -- LINE9-6_(2)/RConn3
  G3/RConn1 -- BUS3/LConn1
  G3/RConn2 -- BUS3/LConn2
  BUS3/LConn3 -- G3/RConn3
  230/13.8/LConn3 -- BUS3/RConn3
  230/13.8/LConn2 -- BUS3/RConn2
  230/13.8/LConn1 -- BUS3/RConn1
  - 89 +/LConn1 -- BUS9/RConn1 -- + 96 -/LConn1
  - 89 +/LConn2 -- + 96 -/LConn2 -- BUS9/RConn2
  - 89 +/LConn3 -- + 96 -/LConn3 -- BUS9/RConn3
  BUS9/LConn1 -- 230/13.8/RConn1
  BUS9/LConn2 -- 230/13.8/RConn2
  BUS9/LConn3 -- 230/13.8/RConn3
